simulink model "ae3e4"  (R2022a)
settings: Solver=VariableStepAuto  StartTime=0.0  StopTime=10.0  RelTol=1e-3
undefined symbols (not defined in the file): sigbuilder_block
settings Model: Creator=attit  LastModifiedBy=attit

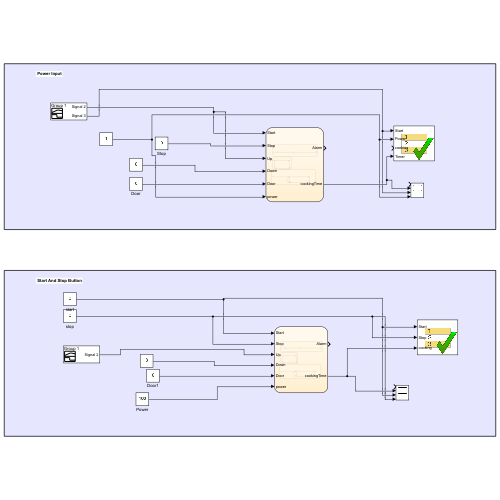
[thumbnail: Simulink's stored preview of the top-level diagram]
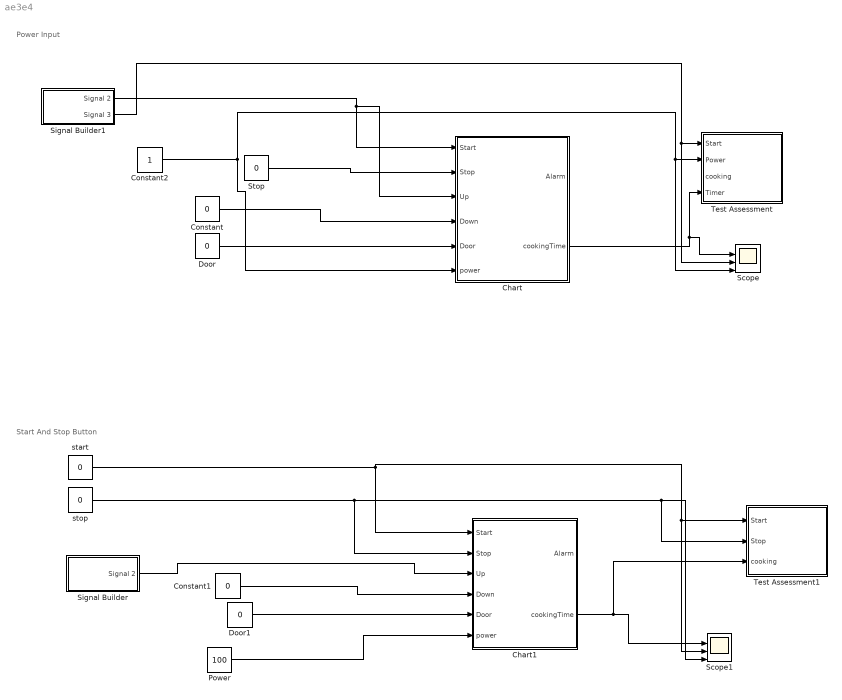
== system ae3e4 ==
  note: Start And Stop Button
  note: Power Input
  Chart : Stateflow chart  TreatAsAtomicUnit=on
  Chart1 : Stateflow chart  TreatAsAtomicUnit=on
  Constant : Constant  Value=0  OutDataTypeStr=boolean
  Constant1 : Constant  Value=0  OutDataTypeStr=boolean
  Constant2 : Constant
  Door : Constant  Value=0  OutDataTypeStr=boolean
  Door1 : Constant  Value=0  OutDataTypeStr=boolean
  Power : Constant  Value=100
  Scope : Scope  NumInputPorts=4
  Scope1 : Scope  NumInputPorts=4
  Signal Builder : Subsystem  Tag=STV Subsys  LoadFcn=sigbuilder_block('load');  StartFcn=sigbuilder_block('start');  StopFcn=sigbuilder_block('stop');  ClipboardFcn=sigbuilder_block('clipboard');  mask(Sigbuilder block){tuvar=[0:10]}
      mask help: Simulink:masks:SigbuilderBlock_MD
      mask init:
      | if ~strcmp(get_param(bdroot(gcbh),'SimulationStatus'),'stopped') tuvar = sigbuilder_block('maskInit'); end
      settings: CopyFcn=sigbuilder_block('copy');  DeleteFcn=sigbuilder_block('delete');  ModelCloseFcn=sigbuilder_block('modelClose');  PreSaveFcn=sigbuilder_block('preSave');  PauseFcn=sigbuilder_block('pause');  ContinueFcn=sigbuilder_block('continue');  NameChangeFcn=sigbuilder_block('namechange');  OpenFcn=sigbuilder_block('open',[437.6 199.2 550.4 400 ]);  CloseFcn=sigbuilder_block('close');
      mask Display: plot(0, 0, 100, 100,[2, 2, 32, 32, 2], [68, 8, 8, 68, 68],[32, 2], [38, 38], [32, 19, 2],[53, 60, 44], [32, 17, 17, 2],[16, 16, 31, 31]);txt = getActiveGroup(gcbh);text(2, 100, txt,'verticalAlignment', 'top');
  Signal Builder1 : Subsystem  Tag=STV Subsys  LoadFcn=sigbuilder_block('load');  StartFcn=sigbuilder_block('start');  StopFcn=sigbuilder_block('stop');  ClipboardFcn=sigbuilder_block('clipboard');  mask(Sigbuilder block){tuvar=[0:10]}
      mask help: Simulink:masks:SigbuilderBlock_MD
      mask init:
      | if ~strcmp(get_param(bdroot(gcbh),'SimulationStatus'),'stopped') tuvar = sigbuilder_block('maskInit'); end
      settings: CopyFcn=sigbuilder_block('copy');  DeleteFcn=sigbuilder_block('delete');  ModelCloseFcn=sigbuilder_block('modelClose');  PreSaveFcn=sigbuilder_block('preSave');  PauseFcn=sigbuilder_block('pause');  ContinueFcn=sigbuilder_block('continue');  NameChangeFcn=sigbuilder_block('namechange');  OpenFcn=sigbuilder_block('open',[437.6 199.2 550.4 400 ]);  CloseFcn=sigbuilder_block('close');
      mask Display: plot(0, 0, 100, 100,[2, 2, 32, 32, 2], [68, 8, 8, 68, 68],[32, 2], [38, 38], [32, 19, 2],[53, 60, 44], [32, 17, 17, 2],[16, 16, 31, 31]);txt = getActiveGroup(gcbh);text(2, 100, txt,'verticalAlignment', 'top');
  Stop : Constant  Value=0  OutDataTypeStr=boolean
  Test Assessment : Test Sequence  TreatAsAtomicUnit=on
  Test Assessment1 : Test Sequence  TreatAsAtomicUnit=on
  start : Constant  Value=0  OutDataTypeStr=boolean
  stop : Constant  Value=0  OutDataTypeStr=boolean
  wires:
  Constant1/1 -> Chart1/4(Down)
  Chart/2(cookingTime) -> Scope/2, Test Assessment/4(Timer)
  Chart1/2(cookingTime) -> Test Assessment1/3(cooking), Scope1/2
  Constant2/1 -> Chart/6(power), Scope/4, Test Assessment/2(Power)
  Power/1 -> Chart1/6(power)
  stop/1 -> Chart1/2(Stop), Test Assessment1/2(Stop), Scope1/4
  Signal Builder1/2(Signal 3) -> Test Assessment/1(Start), Scope/3
  Signal Builder1/1(Signal 2) -> Chart/1(Start), Chart/3(Up)
  Stop/1 -> Chart/2(Stop)
  Constant/1 -> Chart/4(Down)
  Door/1 -> Chart/5(Door)
  start/1 -> Scope1/3, Test Assessment1/1(Start), Chart1/1(Start)
  Door1/1 -> Chart1/5(Door)
  Signal Builder/1(Signal 2) -> Chart1/3(Up)

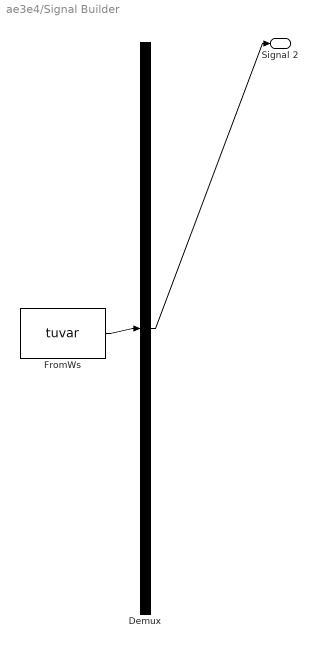
== system ae3e4/Signal Builder ==
  Demux : Demux  Tag=STV Demux  Outputs=1
      settings: DisplayOption=none
  FromWs : FromWorkspace  Tag=STV FromWs  VariableName=tuvar
      SigBuilderData=|
      | common.afterFinalStr = 'Extrapolate'
      | common.sampleTime = 0
      | dataSet.timeRange = [0 10]
      | dataSet.name = 'Group 1'
      | sbobj.Groups.Name = 'Group 1'
      | sbobj.Groups.Signals.Name = 'Signal 2'
      | sbobj.Groups.Signals.XData = [0 5 5 10]
      | sbobj.Groups.Signals.YData = [0 0 1 1]
  Signal 2 : Outport  Tag=STV Outport
  wires:
  Demux/1 -> Signal 2/1
  FromWs/1 -> Demux/1

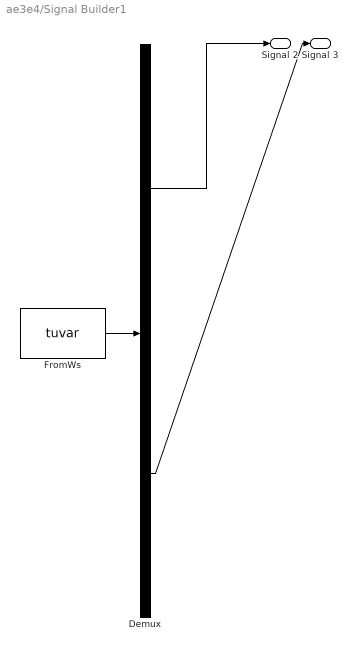
== system ae3e4/Signal Builder1 ==
  Demux : Demux  Tag=STV Demux  Outputs=2
      settings: DisplayOption=none
  FromWs : FromWorkspace  Tag=STV FromWs  VariableName=tuvar
      SigBuilderData=|
      | common.afterFinalStr = 'Extrapolate'
      | common.sampleTime = 0
      | dataSet.timeRange = [0 10]
      | dataSet.name = 'Group 1'
      | sbobj.Groups.Name = 'Group 1'
      | sbobj.Groups.Signals(1).Name = 'Signal 2'
      | sbobj.Groups.Signals(1).XData = [0 3.02 3.02 10]
      | sbobj.Groups.Signals(1).YData = [0 0 1 1]
      | sbobj.Groups.Signals(2).Name = 'Signal 3'
      | sbobj.Groups.Signals(2).XData = [0 7.02 7.02 10]
      | sbobj.Groups.Signals(2).YData = [0 0 1 1]
  Signal 2 : Outport  Tag=STV Outport
  Signal 3 : Outport  Tag=STV Outport  Port=2
  wires:
  FromWs/1 -> Demux/1
  Demux/1 -> Signal 2/1
  Demux/2 -> Signal 3/1

== stateflow chart ae3e4/Test Assessment ==
  state Sl_1
    state step_1
      a=true;
    state step_2
      if(Timer>0)
      a=(cooking<1);
      else
      a=true;
      end
      verify(a,'Sl no.1');
    (default) -> Sl_1.step_1
    Sl_1.step_1 -> Sl_1.step_2 : [
        | Timer>0&&(abs(Power-0)<0.001)&&Start>0
        | ]
  state Sl_2
    state step_1
      a=true;
    state step_2
      if(Timer>0)
      a=(abs(cooking-1)<0.001);
      else
      a=true;
      end
      verify(a,'Sl no.2');
    (default) -> Sl_2.step_1
    Sl_2.step_1 -> Sl_2.step_2 : [
        | Timer>0&&Power>0&&Start>0
        | ]
  state Sl_3
    state step_1
      a=true;
    state step_2
      if(Timer>0)
      a=(abs(cooking-1)<0.001);
      else
      a=true;
      end
      verify(a,'Sl no.3');
    state step_3
      if(Timer>0)
      a=(abs(cooking-0)<0.001);
      else
      a=true;
      end
      verify(a,'Sl no.3');
    (default) -> Sl_3.step_1
    Sl_3.step_1 -> Sl_3.step_2 : [
        | Timer>0&&Power>0&&Start>0
        | ]
    Sl_3.step_2 -> step_3 : [
        | abs(Power-0)<0.001
        | ]
  (default) -> Sl_1 [order 1] : [Active_Scenario_Index == 1]
  (default) -> Sl_2 [order 2] : [Active_Scenario_Index == 2]
  (default) -> Sl_3 [order 3] : {assert(Active_Scenario_Index == 3,'The value of Scenario Parameter ''Active_Scenario_Index'' is not valid. Use the index of the scenario to specify it.')}
  data: Start input; Power input; cooking input; Timer input; Active_Scenario_Index parameter =2; a local

== stateflow chart ae3e4/Chart1 ==
  state oven [parallel]
    du:
    ticks=mod(ticks+1,11)
    settings: executionOrder=1
    oven -> (junction 437)
    (junction 437) -> (junction 441) : [ticks >=10&&cooking==true]
        | {cookingTime=cookingTime-1;
        | ticks = 0;}
    (junction 441) -> (junction 554) : [cooking==true&&cookingTime==0]{Alarm=true}
  state Oven [parallel]
    en,du:
    settings: executionOrder=2
    Oven -> (junction 251)
    (junction 251) -> (junction 257) [order 1] : [Up==1]
        | {cookingTime=cookingTime+30}
    (junction 251) -> (junction 255) [order 2] : [Down==1]
        | {cookingTime=cookingTime-30}
    (junction 257) -> (junction 263)
    (junction 263) -> (junction 255)
  state Cooking [parallel]
    du:
    settings: executionOrder=3
    Cooking -> (junction 279)
    (junction 279) -> (junction 297) [order 1] : [Door==0&&Start==1]{cooking=true;
        | cookingTime;}
    (junction 279) -> (junction 283) [order 3] : [Door==1]{cooking=false;
        | cookingTime=cookingTime-1}
    (junction 279) -> (junction 283) [order 2] : [Door==0&&Stop==1]
        | {cooking=false;
        | cookingTime==cookingTime-1;Alarm=false;}
    (junction 297) -> (junction 299)
    (junction 299) -> (junction 283)
  data: Start input boolean; Stop input boolean; Up input double; Down input boolean; Alarm output boolean =false; Door input boolean; cooking local boolean =false; cookingTime output uint16 [0..] =uint16(0); ticks local uint16 =uint16(0); power input

== stateflow chart ae3e4/Chart ==
  state oven [parallel]
    du:
    ticks=mod(ticks+1,11)
    settings: executionOrder=1
    oven -> (junction 437)
    (junction 437) -> (junction 441) : [ticks >=10&&cooking==true]
        | {cookingTime=cookingTime-1;
        | ticks = 0;}
    (junction 441) -> (junction 554) : [cooking==true&&cookingTime==0]{Alarm=true}
  state Oven [parallel]
    en,du:
    settings: executionOrder=2
    Oven -> (junction 251)
    (junction 251) -> (junction 257) [order 1] : [Up==1]
        | {cookingTime=cookingTime+30}
    (junction 251) -> (junction 255) [order 2] : [Down==1]
        | {cookingTime=cookingTime-30}
    (junction 257) -> (junction 263)
    (junction 263) -> (junction 255)
  state Cooking [parallel]
    du:
    settings: executionOrder=3
    Cooking -> (junction 279)
    (junction 279) -> (junction 297) [order 1] : [Door==0&&Start==1]{cooking=true;
        | cookingTime;}
    (junction 279) -> (junction 283) [order 3] : [Door==1]{cooking=false;
        | cookingTime=cookingTime-1}
    (junction 279) -> (junction 283) [order 2] : [Door==0&&Stop==1]
        | {cooking=false;
        | cookingTime==cookingTime-1;Alarm=false;}
    (junction 297) -> (junction 299)
    (junction 299) -> (junction 283)
  data: Start input double; Stop input boolean; Up input double; Down input boolean; Alarm output boolean =false; Door input boolean; cooking local boolean =false; cookingTime output uint16 [0..] =uint16(0); ticks local uint16 =uint16(0); power input

== stateflow chart ae3e4/Test Assessment1 ==
  state SL_4
    state Step1
      if(Start>0)
      a=(cooking<1);
      else
      a=true;
      end
      verify(a,'Sl no.4');
      settings: description=Sl no. 4
    (default) -> Step1
  state Sl_5
    state Step0
      if(Start>0)
      a=(cooking>0);
      else
      a=true;
      end
      verify(a,'Sl no.5');
    state step_1
      a=true;
    (default) -> Sl_5.Step0
    Sl_5.Step0 -> Sl_5.step_1 : [
        | after(60,sec)
        | ]
  state Sl_6
    state Step0
      if(Start>0)
      a=(cooking>0);
      else
      a=true;
      end
      verify(a,'Sl no.6');
    state step_1
      if(Stop>0)
      a=(cooking~=1);
      else
      a=true;
      end
      verify(a,'Sl no.6');
    state step_2
      a=true;
    (default) -> Sl_6.Step0
    Sl_6.Step0 -> Sl_6.step_1 : [
        | after(2,sec)
        | ]
    Sl_6.step_1 -> Sl_6.step_2 : [
        | after(300,sec)
        | ]
  state Sl_7
    state Step0
      if(Start>0)
      a=(cooking>0);
      else
      a=true;
      end
      verify(a,'Sl no.7');
    state step_1
      if(Stop>0)
      a=(cooking~=1);
      else
      a=true;
      end
      verify(a,'Sl no.7');
    state step_2
      a=true;
      if(Start>0)
      a=(cooking>0);
      else
      a=true;
      end
      verify(a,'Sl no.7');
    state step_3
      a=true;
    (default) -> Sl_7.Step0
    Sl_7.Step0 -> Sl_7.step_1 : [
        | after(2,sec)
        | ]
    Sl_7.step_1 -> Sl_7.step_2 : [
        | after(2,sec)
        | ]
    Sl_7.step_2 -> step_3 : [
        | after(50,sec)
        | ]
  state Sl_8
    state Step0
      if(Start>0)
      a=(cooking>0);
      else
      a=true;
      end
      verify(a,'Sl no.8');
    state step_1
      if(Stop>0)
      a=(cooking~=1);
      else
      a=true;
      end
      verify(a,'Sl no.8');
    state step_2
      a=true;
      a=(abs(cooking-0)<0.001);
      verify(a,'Sl no.8');
    (default) -> Sl_8.Step0
    Sl_8.Step0 -> Sl_8.step_1 : [
        | after(2,sec)
        | ]
    Sl_8.step_1 -> Sl_8.step_2 : [
        | after(300,sec)
        | ]
  (default) -> SL_4 [order 1] : [Active_Scenario_Index == 1]
  (default) -> Sl_5 [order 2] : [Active_Scenario_Index == 2]
  (default) -> Sl_6 [order 3] : [Active_Scenario_Index == 3]
  (default) -> Sl_7 [order 4] : [Active_Scenario_Index == 4]
  (default) -> Sl_8 [order 5] : {assert(Active_Scenario_Index == 5,'The value of Scenario Parameter ''Active_Scenario_Index'' is not valid. Use the index of the scenario to specify it.')}
  data: Start input; Stop input; cooking input; Active_Scenario_Index parameter =1; a local
